simulink model "TST_AccPed_DoCoordOut"  (R2016b)
settings: Solver=FixedStepDiscrete  StartTime=0.0  StopTime=simTime  FixedStep=sampleTime  RelTol=1e-3
values from neighbouring files (symbols this model uses):
  testCase = 1    [initTST_AccPed_DoCoordOut_001.m]    (also in initTST_AccPed_DoCoordOut_002.m = 2; initTST_AccPed_DoCoordOut_003.m = 3)
libraries: simulink x31, UnitTest_Lib x27
settings Model: Creator=zhengjinyan  LastModifiedBy=zhengjinyan
settings DebuggingCC: SignalRangeChecking=error

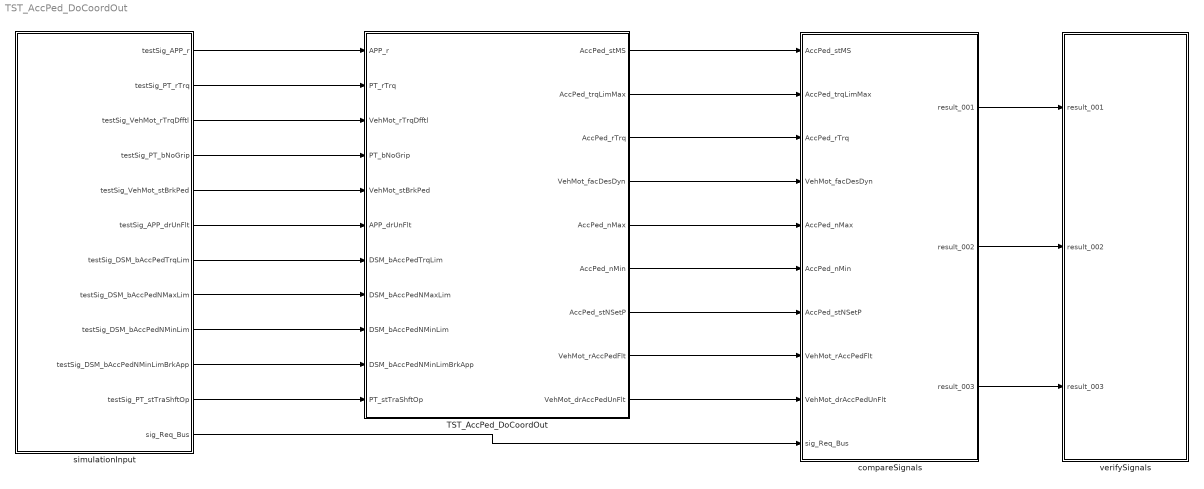
== system TST_AccPed_DoCoordOut ==
  TST_AccPed_DoCoordOut : Subsystem
  compareSignals : Subsystem
  simulationInput : Subsystem
  verifySignals : Subsystem
  wires:
  simulationInput/1(testSig_APP_r) -> TST_AccPed_DoCoordOut/1(APP_r)
  simulationInput/2(testSig_PT_rTrq) -> TST_AccPed_DoCoordOut/2(PT_rTrq)
  simulationInput/3(testSig_VehMot_rTrqDfftl) -> TST_AccPed_DoCoordOut/3(VehMot_rTrqDfftl)
  simulationInput/4(testSig_PT_bNoGrip) -> TST_AccPed_DoCoordOut/4(PT_bNoGrip)
  simulationInput/5(testSig_VehMot_stBrkPed) -> TST_AccPed_DoCoordOut/5(VehMot_stBrkPed)
  simulationInput/6(testSig_APP_drUnFlt) -> TST_AccPed_DoCoordOut/6(APP_drUnFlt)
  simulationInput/7(testSig_DSM_bAccPedTrqLim) -> TST_AccPed_DoCoordOut/7(DSM_bAccPedTrqLim)
  simulationInput/8(testSig_DSM_bAccPedNMaxLim) -> TST_AccPed_DoCoordOut/8(DSM_bAccPedNMaxLim)
  simulationInput/9(testSig_DSM_bAccPedNMinLim) -> TST_AccPed_DoCoordOut/9(DSM_bAccPedNMinLim)
  simulationInput/10(testSig_DSM_bAccPedNMinLimBrkApp) -> TST_AccPed_DoCoordOut/10(DSM_bAccPedNMinLimBrkApp)
  simulationInput/11(testSig_PT_stTraShftOp) -> TST_AccPed_DoCoordOut/11(PT_stTraShftOp)
  TST_AccPed_DoCoordOut/1(AccPed_stMS) -> compareSignals/1(AccPed_stMS)
  TST_AccPed_DoCoordOut/2(AccPed_trqLimMax) -> compareSignals/2(AccPed_trqLimMax)
  TST_AccPed_DoCoordOut/3(AccPed_rTrq) -> compareSignals/3(AccPed_rTrq)
  TST_AccPed_DoCoordOut/4(VehMot_facDesDyn) -> compareSignals/4(VehMot_facDesDyn)
  TST_AccPed_DoCoordOut/5(AccPed_nMax) -> compareSignals/5(AccPed_nMax)
  TST_AccPed_DoCoordOut/6(AccPed_nMin) -> compareSignals/6(AccPed_nMin)
  TST_AccPed_DoCoordOut/7(AccPed_stNSetP) -> compareSignals/7(AccPed_stNSetP)
  TST_AccPed_DoCoordOut/8(VehMot_rAccPedFlt) -> compareSignals/8(VehMot_rAccPedFlt)
  TST_AccPed_DoCoordOut/9(VehMot_drAccPedUnFlt) -> compareSignals/9(VehMot_drAccPedUnFlt)
  simulationInput/12(sig_Req_Bus) -> compareSignals/10(sig_Req_Bus)
  compareSignals/1(result_001) -> verifySignals/1(result_001)
  compareSignals/2(result_002) -> verifySignals/2(result_002)
  compareSignals/3(result_003) -> verifySignals/3(result_003)

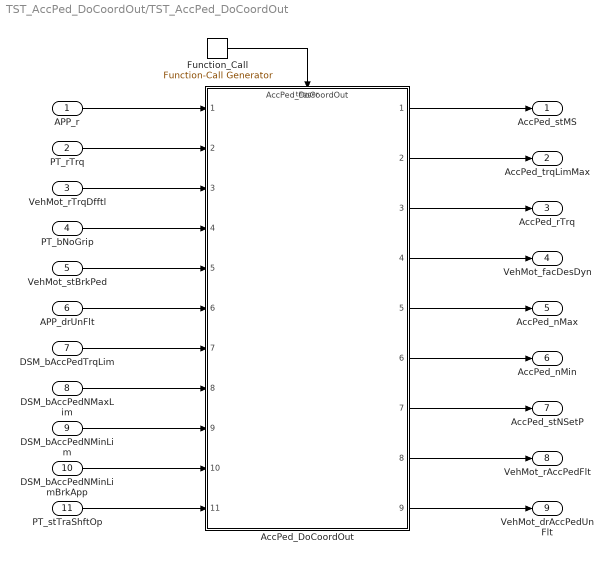
== system TST_AccPed_DoCoordOut/TST_AccPed_DoCoordOut ==
  APP_r : Inport
  PT_rTrq : Inport  Port=2
  VehMot_rTrqDfftl : Inport  Port=3
  PT_bNoGrip : Inport  Port=4
  VehMot_stBrkPed : Inport  Port=5
  APP_drUnFlt : Inport  Port=6
  DSM_bAccPedTrqLim : Inport  Port=7
  DSM_bAccPedNMaxLim : Inport  Port=8
  DSM_bAccPedNMinLim : Inport  Port=9
  DSM_bAccPedNMinLimBrkApp : Inport  Port=10
  PT_stTraShftOp : Inport  Port=11
  AccPed_DoCoordOut : ModelReference  ModelNameDialog=AccPed_DoCoordOut  SimulationMode=Normal  ModelReferenceVersion=1.27  TriggerPortName=function  TriggerPortTriggerType=function-call  TriggerPortStatesWhenEnabling=held
  Function_Call : simulink/Ports & Subsystems/Function-Call Generator  sample_time=sampleTime  numberOfIterations=1
  AccPed_stMS : Outport
  AccPed_trqLimMax : Outport  Port=2
  AccPed_rTrq : Outport  Port=3
  VehMot_facDesDyn : Outport  Port=4
  AccPed_nMax : Outport  Port=5
  AccPed_nMin : Outport  Port=6
  AccPed_stNSetP : Outport  Port=7
  VehMot_rAccPedFlt : Outport  Port=8
  VehMot_drAccPedUnFlt : Outport  Port=9
  wires:
  Function_Call/1 -> AccPed_DoCoordOut/Trigger
  APP_r/1 -> AccPed_DoCoordOut/1
  PT_rTrq/1 -> AccPed_DoCoordOut/2
  VehMot_rTrqDfftl/1 -> AccPed_DoCoordOut/3
  PT_bNoGrip/1 -> AccPed_DoCoordOut/4
  VehMot_stBrkPed/1 -> AccPed_DoCoordOut/5
  APP_drUnFlt/1 -> AccPed_DoCoordOut/6
  DSM_bAccPedTrqLim/1 -> AccPed_DoCoordOut/7
  DSM_bAccPedNMaxLim/1 -> AccPed_DoCoordOut/8
  DSM_bAccPedNMinLim/1 -> AccPed_DoCoordOut/9
  DSM_bAccPedNMinLimBrkApp/1 -> AccPed_DoCoordOut/10
  PT_stTraShftOp/1 -> AccPed_DoCoordOut/11
  AccPed_DoCoordOut/1 -> AccPed_stMS/1
  AccPed_DoCoordOut/2 -> AccPed_trqLimMax/1
  AccPed_DoCoordOut/3 -> AccPed_rTrq/1
  AccPed_DoCoordOut/4 -> VehMot_facDesDyn/1
  AccPed_DoCoordOut/5 -> AccPed_nMax/1
  AccPed_DoCoordOut/6 -> AccPed_nMin/1
  AccPed_DoCoordOut/7 -> AccPed_stNSetP/1
  AccPed_DoCoordOut/8 -> VehMot_rAccPedFlt/1
  AccPed_DoCoordOut/9 -> VehMot_drAccPedUnFlt/1

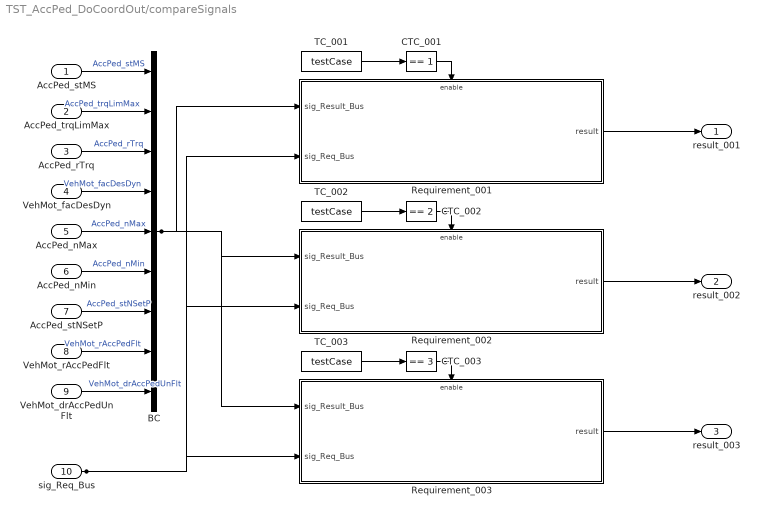
== system TST_AccPed_DoCoordOut/compareSignals ==
  AccPed_stMS : Inport
  AccPed_trqLimMax : Inport  Port=2
  AccPed_rTrq : Inport  Port=3
  VehMot_facDesDyn : Inport  Port=4
  AccPed_nMax : Inport  Port=5
  AccPed_nMin : Inport  Port=6
  AccPed_stNSetP : Inport  Port=7
  VehMot_rAccPedFlt : Inport  Port=8
  VehMot_drAccPedUnFlt : Inport  Port=9
  sig_Req_Bus : Inport  Port=10
  BC : BusCreator  Inputs=9
  CTC_001 : simulink/Logic and Bit Operations/Compare To Constant  relop===  const=1  OutDataTypeStr=boolean
  CTC_002 : simulink/Logic and Bit Operations/Compare To Constant  relop===  const=2  OutDataTypeStr=boolean
  CTC_003 : simulink/Logic and Bit Operations/Compare To Constant  relop===  const=3  OutDataTypeStr=boolean
  Requirement_001 : Subsystem
  Requirement_002 : Subsystem
  Requirement_003 : Subsystem
  TC_001 : Constant  Value=testCase
  TC_002 : Constant  Value=testCase
  TC_003 : Constant  Value=testCase
  result_001 : Outport
  result_002 : Outport  Port=2
  result_003 : Outport  Port=3
  wires:
  AccPed_stMS/1 -> BC/1  "AccPed_stMS"
  AccPed_trqLimMax/1 -> BC/2  "AccPed_trqLimMax"
  AccPed_rTrq/1 -> BC/3  "AccPed_rTrq"
  VehMot_facDesDyn/1 -> BC/4  "VehMot_facDesDyn"
  AccPed_nMax/1 -> BC/5  "AccPed_nMax"
  AccPed_nMin/1 -> BC/6  "AccPed_nMin"
  AccPed_stNSetP/1 -> BC/7  "AccPed_stNSetP"
  VehMot_rAccPedFlt/1 -> BC/8  "VehMot_rAccPedFlt"
  VehMot_drAccPedUnFlt/1 -> BC/9  "VehMot_drAccPedUnFlt"
  TC_001/1 -> CTC_001/1
  CTC_001/1 -> Requirement_001/Enable
  sig_Req_Bus/1 -> Requirement_001/2(sig_Req_Bus), Requirement_002/2(sig_Req_Bus), Requirement_003/2(sig_Req_Bus)
  BC/1 -> Requirement_001/1(sig_Result_Bus), Requirement_002/1(sig_Result_Bus), Requirement_003/1(sig_Result_Bus)
  Requirement_001/1(result) -> result_001/1
  TC_002/1 -> CTC_002/1
  CTC_002/1 -> Requirement_002/Enable
  Requirement_002/1(result) -> result_002/1
  TC_003/1 -> CTC_003/1
  CTC_003/1 -> Requirement_003/Enable
  Requirement_003/1(result) -> result_003/1

== system TST_AccPed_DoCoordOut/simulationInput ==
  BS : BusSelector  OutputSignals=testSig_APP_r,testSig_PT_rTrq,testSig_VehMot_rTrqDfftl,testSig_PT_bNoGrip,testSig_VehMot_stBrkPed,testSig_APP_drUnFlt,testSig_DSM_bAccPedTrqLim,testSig_DSM_bAccPedNMaxLim,testSig_DSM_bAccPedNMinLim,testSig_DSM_bAccPedNMinLimBrkApp,testSig_PT_stTraShftOp
  MPSw : MultiPortSwitch  SaturateOnIntegerOverflow=on  InputSameDT=on
  TestCase : Constant  Value=testCase
  testSignals_R001 : Subsystem
  testSignals_R002 : Subsystem
  testSignals_R003 : Subsystem
  testSig_APP_r : Outport
  testSig_PT_rTrq : Outport  Port=2
  testSig_VehMot_rTrqDfftl : Outport  Port=3
  testSig_PT_bNoGrip : Outport  Port=4
  testSig_VehMot_stBrkPed : Outport  Port=5
  testSig_APP_drUnFlt : Outport  Port=6
  testSig_DSM_bAccPedTrqLim : Outport  Port=7
  testSig_DSM_bAccPedNMaxLim : Outport  Port=8
  testSig_DSM_bAccPedNMinLim : Outport  Port=9
  testSig_DSM_bAccPedNMinLimBrkApp : Outport  Port=10
  testSig_PT_stTraShftOp : Outport  Port=11
  sig_Req_Bus : Outport  Port=12
  wires:
  BS/1 -> testSig_APP_r/1  "<testSig_APP_r>"
  BS/2 -> testSig_PT_rTrq/1  "<testSig_PT_rTrq>"
  BS/3 -> testSig_VehMot_rTrqDfftl/1  "<testSig_VehMot_rTrqDfftl>"
  BS/4 -> testSig_PT_bNoGrip/1  "<testSig_PT_bNoGrip>"
  BS/5 -> testSig_VehMot_stBrkPed/1  "<testSig_VehMot_stBrkPed>"
  BS/6 -> testSig_APP_drUnFlt/1  "<testSig_APP_drUnFlt>"
  BS/7 -> testSig_DSM_bAccPedTrqLim/1  "<testSig_DSM_bAccPedTrqLim>"
  BS/8 -> testSig_DSM_bAccPedNMaxLim/1  "<testSig_DSM_bAccPedNMaxLim>"
  BS/9 -> testSig_DSM_bAccPedNMinLim/1  "<testSig_DSM_bAccPedNMinLim>"
  BS/10 -> testSig_DSM_bAccPedNMinLimBrkApp/1  "<testSig_DSM_bAccPedNMinLimBrkApp>"
  BS/11 -> testSig_PT_stTraShftOp/1  "<testSig_PT_stTraShftOp>"
  MPSw/1 -> BS/1, sig_Req_Bus/1
  TestCase/1 -> MPSw/1
  testSignals_R001/1(testSignals) -> MPSw/2
  testSignals_R002/1(testSignals) -> MPSw/3
  testSignals_R003/1(testSignals) -> MPSw/4

== system TST_AccPed_DoCoordOut/verifySignals ==
  result_001 : Inport
  result_002 : Inport  Port=2
  result_003 : Inport  Port=3
  Assertion_001 : Assertion  Enabled=off
  Assertion_002 : Assertion  Enabled=off
  Assertion_003 : Assertion  Enabled=off
  wires:
  result_001/1 -> Assertion_001/1
  result_002/1 -> Assertion_002/1
  result_003/1 -> Assertion_003/1

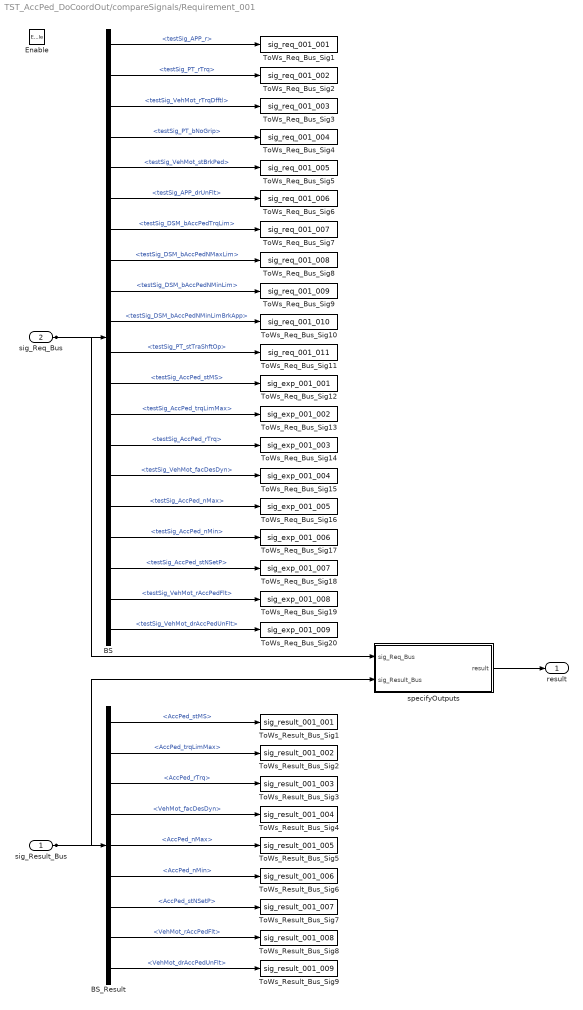
== system TST_AccPed_DoCoordOut/compareSignals/Requirement_001 ==
  sig_Result_Bus : Inport
  sig_Req_Bus : Inport  Port=2
  Enable : EnablePort
  BS : BusSelector  OutputSignals=testSig_APP_r,testSig_PT_rTrq,testSig_VehMot_rTrqDfftl,testSig_PT_bNoGrip,testSig_VehMot_stBrkPed,testSig_APP_drUnFlt,testSig_DSM_bAccPedTrqLim,testSig_DSM_bAccPedNMaxLim,testSig_DSM_bAccPedNMinLim,testSig_DSM_bAccPedNMinLimBrkApp,testSig_PT_stTraShftOp,testSig_AccPed_stMS,testSig_AccPed_trqLimMax,testSig_AccPed_rTrq,testSig_VehMot_facDesDyn,testSig_AccPed_nMax,testSig_AccPed_nMin,testSig_AccPed_stNSetP,testSig_VehMot_rAccPedFlt,testSig_VehMot_drAccPedUnFlt
  BS_Result : BusSelector  OutputSignals=AccPed_stMS,AccPed_trqLimMax,AccPed_rTrq,VehMot_facDesDyn,AccPed_nMax,AccPed_nMin,AccPed_stNSetP,VehMot_rAccPedFlt,VehMot_drAccPedUnFlt
  ToWs_Req_Bus_Sig1 : ToWorkspace  VariableName=sig_req_001_001  SaveFormat=Structure With Time
  ToWs_Req_Bus_Sig10 : ToWorkspace  VariableName=sig_req_001_010  SaveFormat=Structure With Time
  ToWs_Req_Bus_Sig11 : ToWorkspace  VariableName=sig_req_001_011  SaveFormat=Structure With Time
  ToWs_Req_Bus_Sig12 : ToWorkspace  VariableName=sig_exp_001_001  SaveFormat=Structure With Time
  ToWs_Req_Bus_Sig13 : ToWorkspace  VariableName=sig_exp_001_002  SaveFormat=Structure With Time
  ToWs_Req_Bus_Sig14 : ToWorkspace  VariableName=sig_exp_001_003  SaveFormat=Structure With Time
  ToWs_Req_Bus_Sig15 : ToWorkspace  VariableName=sig_exp_001_004  SaveFormat=Structure With Time
  ToWs_Req_Bus_Sig16 : ToWorkspace  VariableName=sig_exp_001_005  SaveFormat=Structure With Time
  ToWs_Req_Bus_Sig17 : ToWorkspace  VariableName=sig_exp_001_006  SaveFormat=Structure With Time
  ToWs_Req_Bus_Sig18 : ToWorkspace  VariableName=sig_exp_001_007  SaveFormat=Structure With Time
  ToWs_Req_Bus_Sig19 : ToWorkspace  VariableName=sig_exp_001_008  SaveFormat=Structure With Time
  ToWs_Req_Bus_Sig2 : ToWorkspace  VariableName=sig_req_001_002  SaveFormat=Structure With Time
  ToWs_Req_Bus_Sig20 : ToWorkspace  VariableName=sig_exp_001_009  SaveFormat=Structure With Time
  ToWs_Req_Bus_Sig3 : ToWorkspace  VariableName=sig_req_001_003  SaveFormat=Structure With Time
  ToWs_Req_Bus_Sig4 : ToWorkspace  VariableName=sig_req_001_004  SaveFormat=Structure With Time
  ToWs_Req_Bus_Sig5 : ToWorkspace  VariableName=sig_req_001_005  SaveFormat=Structure With Time
  ToWs_Req_Bus_Sig6 : ToWorkspace  VariableName=sig_req_001_006  SaveFormat=Structure With Time
  ToWs_Req_Bus_Sig7 : ToWorkspace  VariableName=sig_req_001_007  SaveFormat=Structure With Time
  ToWs_Req_Bus_Sig8 : ToWorkspace  VariableName=sig_req_001_008  SaveFormat=Structure With Time
  ToWs_Req_Bus_Sig9 : ToWorkspace  VariableName=sig_req_001_009  SaveFormat=Structure With Time
  ToWs_Result_Bus_Sig1 : ToWorkspace  VariableName=sig_result_001_001  SaveFormat=Structure With Time
  ToWs_Result_Bus_Sig2 : ToWorkspace  VariableName=sig_result_001_002  SaveFormat=Structure With Time
  ToWs_Result_Bus_Sig3 : ToWorkspace  VariableName=sig_result_001_003  SaveFormat=Structure With Time
  ToWs_Result_Bus_Sig4 : ToWorkspace  VariableName=sig_result_001_004  SaveFormat=Structure With Time
  ToWs_Result_Bus_Sig5 : ToWorkspace  VariableName=sig_result_001_005  SaveFormat=Structure With Time
  ToWs_Result_Bus_Sig6 : ToWorkspace  VariableName=sig_result_001_006  SaveFormat=Structure With Time
  ToWs_Result_Bus_Sig7 : ToWorkspace  VariableName=sig_result_001_007  SaveFormat=Structure With Time
  ToWs_Result_Bus_Sig8 : ToWorkspace  VariableName=sig_result_001_008  SaveFormat=Structure With Time
  ToWs_Result_Bus_Sig9 : ToWorkspace  VariableName=sig_result_001_009  SaveFormat=Structure With Time
  specifyOutputs : Subsystem
  result : Outport
  wires:
  sig_Req_Bus/1 -> BS/1, specifyOutputs/1(sig_Req_Bus)
  BS/1 -> ToWs_Req_Bus_Sig1/1  "<testSig_APP_r>"
  BS/2 -> ToWs_Req_Bus_Sig2/1  "<testSig_PT_rTrq>"
  BS/3 -> ToWs_Req_Bus_Sig3/1  "<testSig_VehMot_rTrqDfftl>"
  BS/4 -> ToWs_Req_Bus_Sig4/1  "<testSig_PT_bNoGrip>"
  BS/5 -> ToWs_Req_Bus_Sig5/1  "<testSig_VehMot_stBrkPed>"
  BS/6 -> ToWs_Req_Bus_Sig6/1  "<testSig_APP_drUnFlt>"
  BS/7 -> ToWs_Req_Bus_Sig7/1  "<testSig_DSM_bAccPedTrqLim>"
  BS/8 -> ToWs_Req_Bus_Sig8/1  "<testSig_DSM_bAccPedNMaxLim>"
  BS/9 -> ToWs_Req_Bus_Sig9/1  "<testSig_DSM_bAccPedNMinLim>"
  BS/10 -> ToWs_Req_Bus_Sig10/1  "<testSig_DSM_bAccPedNMinLimBrkApp>"
  BS/11 -> ToWs_Req_Bus_Sig11/1  "<testSig_PT_stTraShftOp>"
  BS/12 -> ToWs_Req_Bus_Sig12/1  "<testSig_AccPed_stMS>"
  BS/13 -> ToWs_Req_Bus_Sig13/1  "<testSig_AccPed_trqLimMax>"
  BS/14 -> ToWs_Req_Bus_Sig14/1  "<testSig_AccPed_rTrq>"
  BS/15 -> ToWs_Req_Bus_Sig15/1  "<testSig_VehMot_facDesDyn>"
  BS/16 -> ToWs_Req_Bus_Sig16/1  "<testSig_AccPed_nMax>"
  BS/17 -> ToWs_Req_Bus_Sig17/1  "<testSig_AccPed_nMin>"
  BS/18 -> ToWs_Req_Bus_Sig18/1  "<testSig_AccPed_stNSetP>"
  BS/19 -> ToWs_Req_Bus_Sig19/1  "<testSig_VehMot_rAccPedFlt>"
  BS/20 -> ToWs_Req_Bus_Sig20/1  "<testSig_VehMot_drAccPedUnFlt>"
  sig_Result_Bus/1 -> BS_Result/1, specifyOutputs/2(sig_Result_Bus)
  BS_Result/1 -> ToWs_Result_Bus_Sig1/1  "<AccPed_stMS>"
  BS_Result/2 -> ToWs_Result_Bus_Sig2/1  "<AccPed_trqLimMax>"
  BS_Result/3 -> ToWs_Result_Bus_Sig3/1  "<AccPed_rTrq>"
  BS_Result/4 -> ToWs_Result_Bus_Sig4/1  "<VehMot_facDesDyn>"
  BS_Result/5 -> ToWs_Result_Bus_Sig5/1  "<AccPed_nMax>"
  BS_Result/6 -> ToWs_Result_Bus_Sig6/1  "<AccPed_nMin>"
  BS_Result/7 -> ToWs_Result_Bus_Sig7/1  "<AccPed_stNSetP>"
  BS_Result/8 -> ToWs_Result_Bus_Sig8/1  "<VehMot_rAccPedFlt>"
  BS_Result/9 -> ToWs_Result_Bus_Sig9/1  "<VehMot_drAccPedUnFlt>"
  specifyOutputs/1(result) -> result/1

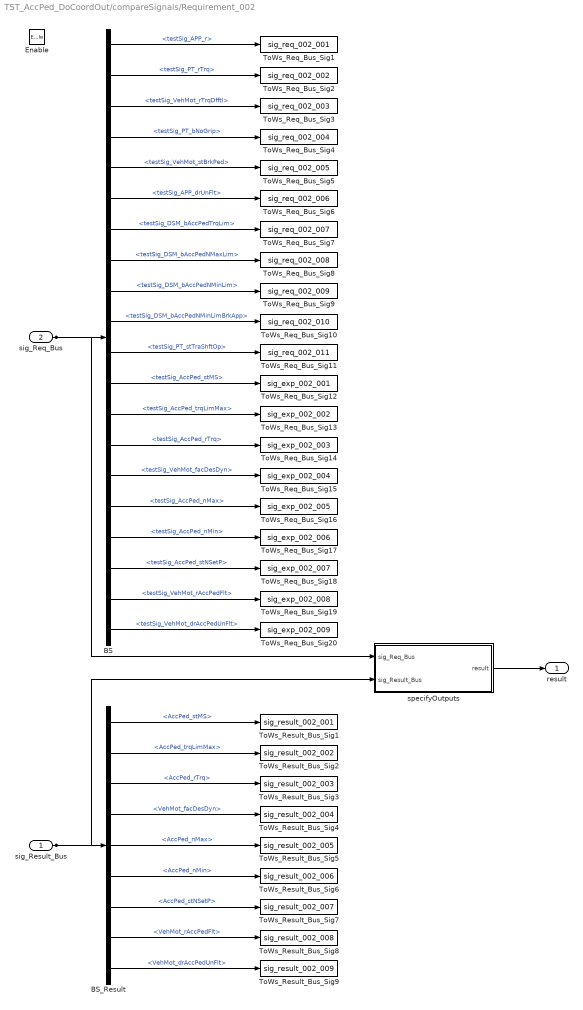
== system TST_AccPed_DoCoordOut/compareSignals/Requirement_002 ==
  sig_Result_Bus : Inport
  sig_Req_Bus : Inport  Port=2
  Enable : EnablePort
  BS : BusSelector  OutputSignals=testSig_APP_r,testSig_PT_rTrq,testSig_VehMot_rTrqDfftl,testSig_PT_bNoGrip,testSig_VehMot_stBrkPed,testSig_APP_drUnFlt,testSig_DSM_bAccPedTrqLim,testSig_DSM_bAccPedNMaxLim,testSig_DSM_bAccPedNMinLim,testSig_DSM_bAccPedNMinLimBrkApp,testSig_PT_stTraShftOp,testSig_AccPed_stMS,testSig_AccPed_trqLimMax,testSig_AccPed_rTrq,testSig_VehMot_facDesDyn,testSig_AccPed_nMax,testSig_AccPed_nMin,testSig_AccPed_stNSetP,testSig_VehMot_rAccPedFlt,testSig_VehMot_drAccPedUnFlt
  BS_Result : BusSelector  OutputSignals=AccPed_stMS,AccPed_trqLimMax,AccPed_rTrq,VehMot_facDesDyn,AccPed_nMax,AccPed_nMin,AccPed_stNSetP,VehMot_rAccPedFlt,VehMot_drAccPedUnFlt
  ToWs_Req_Bus_Sig1 : ToWorkspace  VariableName=sig_req_002_001  SaveFormat=Structure With Time
  ToWs_Req_Bus_Sig10 : ToWorkspace  VariableName=sig_req_002_010  SaveFormat=Structure With Time
  ToWs_Req_Bus_Sig11 : ToWorkspace  VariableName=sig_req_002_011  SaveFormat=Structure With Time
  ToWs_Req_Bus_Sig12 : ToWorkspace  VariableName=sig_exp_002_001  SaveFormat=Structure With Time
  ToWs_Req_Bus_Sig13 : ToWorkspace  VariableName=sig_exp_002_002  SaveFormat=Structure With Time
  ToWs_Req_Bus_Sig14 : ToWorkspace  VariableName=sig_exp_002_003  SaveFormat=Structure With Time
  ToWs_Req_Bus_Sig15 : ToWorkspace  VariableName=sig_exp_002_004  SaveFormat=Structure With Time
  ToWs_Req_Bus_Sig16 : ToWorkspace  VariableName=sig_exp_002_005  SaveFormat=Structure With Time
  ToWs_Req_Bus_Sig17 : ToWorkspace  VariableName=sig_exp_002_006  SaveFormat=Structure With Time
  ToWs_Req_Bus_Sig18 : ToWorkspace  VariableName=sig_exp_002_007  SaveFormat=Structure With Time
  ToWs_Req_Bus_Sig19 : ToWorkspace  VariableName=sig_exp_002_008  SaveFormat=Structure With Time
  ToWs_Req_Bus_Sig2 : ToWorkspace  VariableName=sig_req_002_002  SaveFormat=Structure With Time
  ToWs_Req_Bus_Sig20 : ToWorkspace  VariableName=sig_exp_002_009  SaveFormat=Structure With Time
  ToWs_Req_Bus_Sig3 : ToWorkspace  VariableName=sig_req_002_003  SaveFormat=Structure With Time
  ToWs_Req_Bus_Sig4 : ToWorkspace  VariableName=sig_req_002_004  SaveFormat=Structure With Time
  ToWs_Req_Bus_Sig5 : ToWorkspace  VariableName=sig_req_002_005  SaveFormat=Structure With Time
  ToWs_Req_Bus_Sig6 : ToWorkspace  VariableName=sig_req_002_006  SaveFormat=Structure With Time
  ToWs_Req_Bus_Sig7 : ToWorkspace  VariableName=sig_req_002_007  SaveFormat=Structure With Time
  ToWs_Req_Bus_Sig8 : ToWorkspace  VariableName=sig_req_002_008  SaveFormat=Structure With Time
  ToWs_Req_Bus_Sig9 : ToWorkspace  VariableName=sig_req_002_009  SaveFormat=Structure With Time
  ToWs_Result_Bus_Sig1 : ToWorkspace  VariableName=sig_result_002_001  SaveFormat=Structure With Time
  ToWs_Result_Bus_Sig2 : ToWorkspace  VariableName=sig_result_002_002  SaveFormat=Structure With Time
  ToWs_Result_Bus_Sig3 : ToWorkspace  VariableName=sig_result_002_003  SaveFormat=Structure With Time
  ToWs_Result_Bus_Sig4 : ToWorkspace  VariableName=sig_result_002_004  SaveFormat=Structure With Time
  ToWs_Result_Bus_Sig5 : ToWorkspace  VariableName=sig_result_002_005  SaveFormat=Structure With Time
  ToWs_Result_Bus_Sig6 : ToWorkspace  VariableName=sig_result_002_006  SaveFormat=Structure With Time
  ToWs_Result_Bus_Sig7 : ToWorkspace  VariableName=sig_result_002_007  SaveFormat=Structure With Time
  ToWs_Result_Bus_Sig8 : ToWorkspace  VariableName=sig_result_002_008  SaveFormat=Structure With Time
  ToWs_Result_Bus_Sig9 : ToWorkspace  VariableName=sig_result_002_009  SaveFormat=Structure With Time
  specifyOutputs : Subsystem
  result : Outport
  wires:
  sig_Req_Bus/1 -> BS/1, specifyOutputs/1(sig_Req_Bus)
  BS/1 -> ToWs_Req_Bus_Sig1/1  "<testSig_APP_r>"
  BS/2 -> ToWs_Req_Bus_Sig2/1  "<testSig_PT_rTrq>"
  BS/3 -> ToWs_Req_Bus_Sig3/1  "<testSig_VehMot_rTrqDfftl>"
  BS/4 -> ToWs_Req_Bus_Sig4/1  "<testSig_PT_bNoGrip>"
  BS/5 -> ToWs_Req_Bus_Sig5/1  "<testSig_VehMot_stBrkPed>"
  BS/6 -> ToWs_Req_Bus_Sig6/1  "<testSig_APP_drUnFlt>"
  BS/7 -> ToWs_Req_Bus_Sig7/1  "<testSig_DSM_bAccPedTrqLim>"
  BS/8 -> ToWs_Req_Bus_Sig8/1  "<testSig_DSM_bAccPedNMaxLim>"
  BS/9 -> ToWs_Req_Bus_Sig9/1  "<testSig_DSM_bAccPedNMinLim>"
  BS/10 -> ToWs_Req_Bus_Sig10/1  "<testSig_DSM_bAccPedNMinLimBrkApp>"
  BS/11 -> ToWs_Req_Bus_Sig11/1  "<testSig_PT_stTraShftOp>"
  BS/12 -> ToWs_Req_Bus_Sig12/1  "<testSig_AccPed_stMS>"
  BS/13 -> ToWs_Req_Bus_Sig13/1  "<testSig_AccPed_trqLimMax>"
  BS/14 -> ToWs_Req_Bus_Sig14/1  "<testSig_AccPed_rTrq>"
  BS/15 -> ToWs_Req_Bus_Sig15/1  "<testSig_VehMot_facDesDyn>"
  BS/16 -> ToWs_Req_Bus_Sig16/1  "<testSig_AccPed_nMax>"
  BS/17 -> ToWs_Req_Bus_Sig17/1  "<testSig_AccPed_nMin>"
  BS/18 -> ToWs_Req_Bus_Sig18/1  "<testSig_AccPed_stNSetP>"
  BS/19 -> ToWs_Req_Bus_Sig19/1  "<testSig_VehMot_rAccPedFlt>"
  BS/20 -> ToWs_Req_Bus_Sig20/1  "<testSig_VehMot_drAccPedUnFlt>"
  sig_Result_Bus/1 -> BS_Result/1, specifyOutputs/2(sig_Result_Bus)
  BS_Result/1 -> ToWs_Result_Bus_Sig1/1  "<AccPed_stMS>"
  BS_Result/2 -> ToWs_Result_Bus_Sig2/1  "<AccPed_trqLimMax>"
  BS_Result/3 -> ToWs_Result_Bus_Sig3/1  "<AccPed_rTrq>"
  BS_Result/4 -> ToWs_Result_Bus_Sig4/1  "<VehMot_facDesDyn>"
  BS_Result/5 -> ToWs_Result_Bus_Sig5/1  "<AccPed_nMax>"
  BS_Result/6 -> ToWs_Result_Bus_Sig6/1  "<AccPed_nMin>"
  BS_Result/7 -> ToWs_Result_Bus_Sig7/1  "<AccPed_stNSetP>"
  BS_Result/8 -> ToWs_Result_Bus_Sig8/1  "<VehMot_rAccPedFlt>"
  BS_Result/9 -> ToWs_Result_Bus_Sig9/1  "<VehMot_drAccPedUnFlt>"
  specifyOutputs/1(result) -> result/1

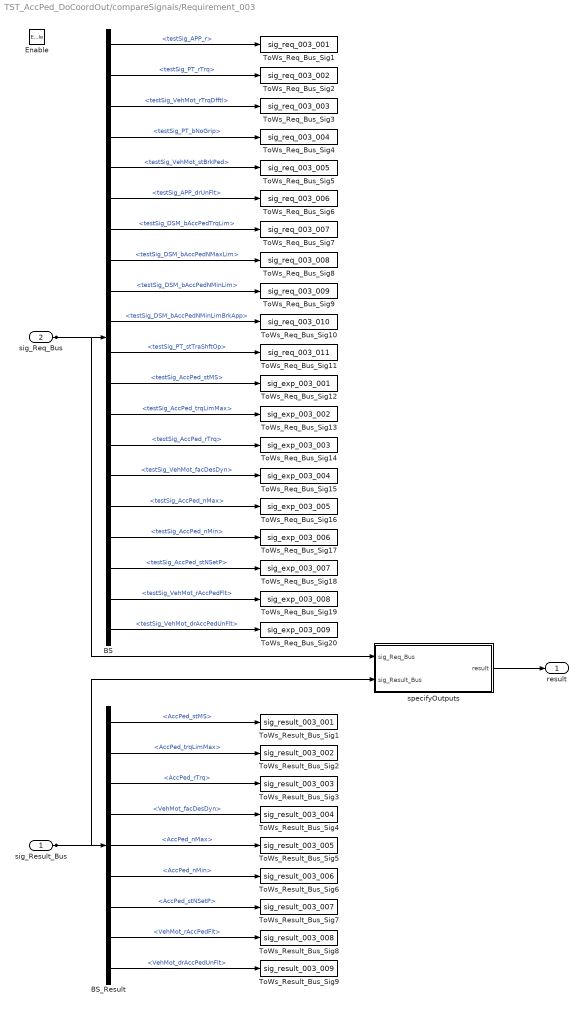
== system TST_AccPed_DoCoordOut/compareSignals/Requirement_003 ==
  sig_Result_Bus : Inport
  sig_Req_Bus : Inport  Port=2
  Enable : EnablePort
  BS : BusSelector  OutputSignals=testSig_APP_r,testSig_PT_rTrq,testSig_VehMot_rTrqDfftl,testSig_PT_bNoGrip,testSig_VehMot_stBrkPed,testSig_APP_drUnFlt,testSig_DSM_bAccPedTrqLim,testSig_DSM_bAccPedNMaxLim,testSig_DSM_bAccPedNMinLim,testSig_DSM_bAccPedNMinLimBrkApp,testSig_PT_stTraShftOp,testSig_AccPed_stMS,testSig_AccPed_trqLimMax,testSig_AccPed_rTrq,testSig_VehMot_facDesDyn,testSig_AccPed_nMax,testSig_AccPed_nMin,testSig_AccPed_stNSetP,testSig_VehMot_rAccPedFlt,testSig_VehMot_drAccPedUnFlt
  BS_Result : BusSelector  OutputSignals=AccPed_stMS,AccPed_trqLimMax,AccPed_rTrq,VehMot_facDesDyn,AccPed_nMax,AccPed_nMin,AccPed_stNSetP,VehMot_rAccPedFlt,VehMot_drAccPedUnFlt
  ToWs_Req_Bus_Sig1 : ToWorkspace  VariableName=sig_req_003_001  SaveFormat=Structure With Time
  ToWs_Req_Bus_Sig10 : ToWorkspace  VariableName=sig_req_003_010  SaveFormat=Structure With Time
  ToWs_Req_Bus_Sig11 : ToWorkspace  VariableName=sig_req_003_011  SaveFormat=Structure With Time
  ToWs_Req_Bus_Sig12 : ToWorkspace  VariableName=sig_exp_003_001  SaveFormat=Structure With Time
  ToWs_Req_Bus_Sig13 : ToWorkspace  VariableName=sig_exp_003_002  SaveFormat=Structure With Time
  ToWs_Req_Bus_Sig14 : ToWorkspace  VariableName=sig_exp_003_003  SaveFormat=Structure With Time
  ToWs_Req_Bus_Sig15 : ToWorkspace  VariableName=sig_exp_003_004  SaveFormat=Structure With Time
  ToWs_Req_Bus_Sig16 : ToWorkspace  VariableName=sig_exp_003_005  SaveFormat=Structure With Time
  ToWs_Req_Bus_Sig17 : ToWorkspace  VariableName=sig_exp_003_006  SaveFormat=Structure With Time
  ToWs_Req_Bus_Sig18 : ToWorkspace  VariableName=sig_exp_003_007  SaveFormat=Structure With Time
  ToWs_Req_Bus_Sig19 : ToWorkspace  VariableName=sig_exp_003_008  SaveFormat=Structure With Time
  ToWs_Req_Bus_Sig2 : ToWorkspace  VariableName=sig_req_003_002  SaveFormat=Structure With Time
  ToWs_Req_Bus_Sig20 : ToWorkspace  VariableName=sig_exp_003_009  SaveFormat=Structure With Time
  ToWs_Req_Bus_Sig3 : ToWorkspace  VariableName=sig_req_003_003  SaveFormat=Structure With Time
  ToWs_Req_Bus_Sig4 : ToWorkspace  VariableName=sig_req_003_004  SaveFormat=Structure With Time
  ToWs_Req_Bus_Sig5 : ToWorkspace  VariableName=sig_req_003_005  SaveFormat=Structure With Time
  ToWs_Req_Bus_Sig6 : ToWorkspace  VariableName=sig_req_003_006  SaveFormat=Structure With Time
  ToWs_Req_Bus_Sig7 : ToWorkspace  VariableName=sig_req_003_007  SaveFormat=Structure With Time
  ToWs_Req_Bus_Sig8 : ToWorkspace  VariableName=sig_req_003_008  SaveFormat=Structure With Time
  ToWs_Req_Bus_Sig9 : ToWorkspace  VariableName=sig_req_003_009  SaveFormat=Structure With Time
  ToWs_Result_Bus_Sig1 : ToWorkspace  VariableName=sig_result_003_001  SaveFormat=Structure With Time
  ToWs_Result_Bus_Sig2 : ToWorkspace  VariableName=sig_result_003_002  SaveFormat=Structure With Time
  ToWs_Result_Bus_Sig3 : ToWorkspace  VariableName=sig_result_003_003  SaveFormat=Structure With Time
  ToWs_Result_Bus_Sig4 : ToWorkspace  VariableName=sig_result_003_004  SaveFormat=Structure With Time
  ToWs_Result_Bus_Sig5 : ToWorkspace  VariableName=sig_result_003_005  SaveFormat=Structure With Time
  ToWs_Result_Bus_Sig6 : ToWorkspace  VariableName=sig_result_003_006  SaveFormat=Structure With Time
  ToWs_Result_Bus_Sig7 : ToWorkspace  VariableName=sig_result_003_007  SaveFormat=Structure With Time
  ToWs_Result_Bus_Sig8 : ToWorkspace  VariableName=sig_result_003_008  SaveFormat=Structure With Time
  ToWs_Result_Bus_Sig9 : ToWorkspace  VariableName=sig_result_003_009  SaveFormat=Structure With Time
  specifyOutputs : Subsystem
  result : Outport
  wires:
  sig_Req_Bus/1 -> BS/1, specifyOutputs/1(sig_Req_Bus)
  BS/1 -> ToWs_Req_Bus_Sig1/1  "<testSig_APP_r>"
  BS/2 -> ToWs_Req_Bus_Sig2/1  "<testSig_PT_rTrq>"
  BS/3 -> ToWs_Req_Bus_Sig3/1  "<testSig_VehMot_rTrqDfftl>"
  BS/4 -> ToWs_Req_Bus_Sig4/1  "<testSig_PT_bNoGrip>"
  BS/5 -> ToWs_Req_Bus_Sig5/1  "<testSig_VehMot_stBrkPed>"
  BS/6 -> ToWs_Req_Bus_Sig6/1  "<testSig_APP_drUnFlt>"
  BS/7 -> ToWs_Req_Bus_Sig7/1  "<testSig_DSM_bAccPedTrqLim>"
  BS/8 -> ToWs_Req_Bus_Sig8/1  "<testSig_DSM_bAccPedNMaxLim>"
  BS/9 -> ToWs_Req_Bus_Sig9/1  "<testSig_DSM_bAccPedNMinLim>"
  BS/10 -> ToWs_Req_Bus_Sig10/1  "<testSig_DSM_bAccPedNMinLimBrkApp>"
  BS/11 -> ToWs_Req_Bus_Sig11/1  "<testSig_PT_stTraShftOp>"
  BS/12 -> ToWs_Req_Bus_Sig12/1  "<testSig_AccPed_stMS>"
  BS/13 -> ToWs_Req_Bus_Sig13/1  "<testSig_AccPed_trqLimMax>"
  BS/14 -> ToWs_Req_Bus_Sig14/1  "<testSig_AccPed_rTrq>"
  BS/15 -> ToWs_Req_Bus_Sig15/1  "<testSig_VehMot_facDesDyn>"
  BS/16 -> ToWs_Req_Bus_Sig16/1  "<testSig_AccPed_nMax>"
  BS/17 -> ToWs_Req_Bus_Sig17/1  "<testSig_AccPed_nMin>"
  BS/18 -> ToWs_Req_Bus_Sig18/1  "<testSig_AccPed_stNSetP>"
  BS/19 -> ToWs_Req_Bus_Sig19/1  "<testSig_VehMot_rAccPedFlt>"
  BS/20 -> ToWs_Req_Bus_Sig20/1  "<testSig_VehMot_drAccPedUnFlt>"
  sig_Result_Bus/1 -> BS_Result/1, specifyOutputs/2(sig_Result_Bus)
  BS_Result/1 -> ToWs_Result_Bus_Sig1/1  "<AccPed_stMS>"
  BS_Result/2 -> ToWs_Result_Bus_Sig2/1  "<AccPed_trqLimMax>"
  BS_Result/3 -> ToWs_Result_Bus_Sig3/1  "<AccPed_rTrq>"
  BS_Result/4 -> ToWs_Result_Bus_Sig4/1  "<VehMot_facDesDyn>"
  BS_Result/5 -> ToWs_Result_Bus_Sig5/1  "<AccPed_nMax>"
  BS_Result/6 -> ToWs_Result_Bus_Sig6/1  "<AccPed_nMin>"
  BS_Result/7 -> ToWs_Result_Bus_Sig7/1  "<AccPed_stNSetP>"
  BS_Result/8 -> ToWs_Result_Bus_Sig8/1  "<VehMot_rAccPedFlt>"
  BS_Result/9 -> ToWs_Result_Bus_Sig9/1  "<VehMot_drAccPedUnFlt>"
  specifyOutputs/1(result) -> result/1

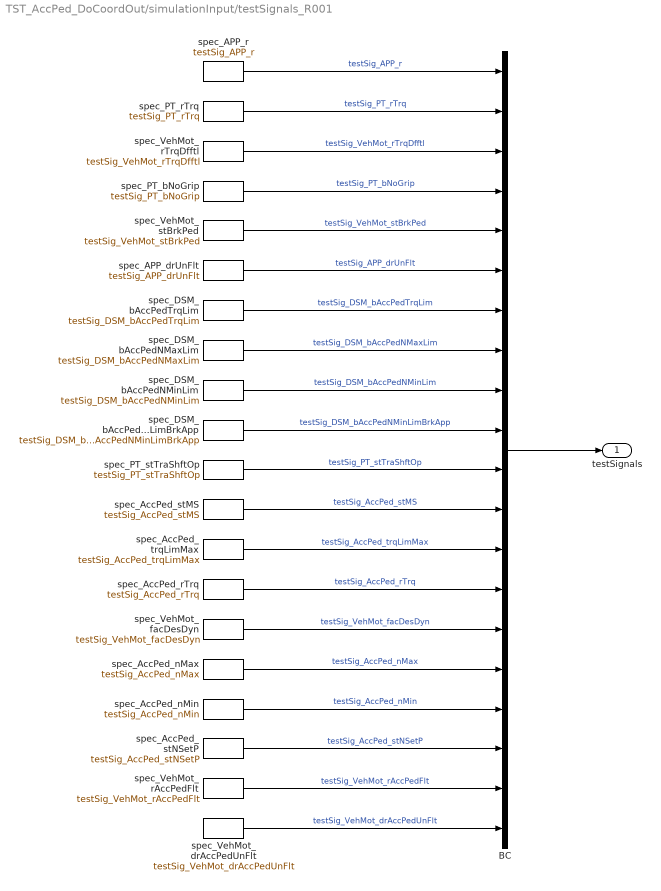
== system TST_AccPed_DoCoordOut/simulationInput/testSignals_R001 ==
  BC : BusCreator  Inputs=20
  spec_APP_drUnFlt : FromWorkspace  VariableName=testSig_APP_drUnFlt  Interpolate=off  OutputAfterFinalValue=Holding final value
  spec_APP_r : FromWorkspace  VariableName=testSig_APP_r  Interpolate=off  OutputAfterFinalValue=Holding final value
  spec_AccPed_nMax : FromWorkspace  VariableName=testSig_AccPed_nMax  Interpolate=off  OutputAfterFinalValue=Holding final value
  spec_AccPed_nMin : FromWorkspace  VariableName=testSig_AccPed_nMin  Interpolate=off  OutputAfterFinalValue=Holding final value
  spec_AccPed_rTrq : FromWorkspace  VariableName=testSig_AccPed_rTrq  Interpolate=off  OutputAfterFinalValue=Holding final value
  spec_AccPed_stMS : FromWorkspace  VariableName=testSig_AccPed_stMS  Interpolate=off  OutputAfterFinalValue=Holding final value
  spec_AccPed_stNSetP : FromWorkspace  VariableName=testSig_AccPed_stNSetP  Interpolate=off  OutputAfterFinalValue=Holding final value
  spec_AccPed_trqLimMax : FromWorkspace  VariableName=testSig_AccPed_trqLimMax  Interpolate=off  OutputAfterFinalValue=Holding final value
  spec_DSM_bAccPedNMaxLim : FromWorkspace  VariableName=testSig_DSM_bAccPedNMaxLim  Interpolate=off  OutputAfterFinalValue=Holding final value
  spec_DSM_bAccPedNMinLim : FromWorkspace  VariableName=testSig_DSM_bAccPedNMinLim  Interpolate=off  OutputAfterFinalValue=Holding final value
  spec_DSM_bAccPedNMinLimBrkApp : FromWorkspace  VariableName=testSig_DSM_bAccPedNMinLimBrkApp  Interpolate=off  OutputAfterFinalValue=Holding final value
  spec_DSM_bAccPedTrqLim : FromWorkspace  VariableName=testSig_DSM_bAccPedTrqLim  Interpolate=off  OutputAfterFinalValue=Holding final value
  spec_PT_bNoGrip : FromWorkspace  VariableName=testSig_PT_bNoGrip  Interpolate=off  OutputAfterFinalValue=Holding final value
  spec_PT_rTrq : FromWorkspace  VariableName=testSig_PT_rTrq  Interpolate=off  OutputAfterFinalValue=Holding final value
  spec_PT_stTraShftOp : FromWorkspace  VariableName=testSig_PT_stTraShftOp  Interpolate=off  OutputAfterFinalValue=Holding final value
  spec_VehMot_drAccPedUnFlt : FromWorkspace  VariableName=testSig_VehMot_drAccPedUnFlt  Interpolate=off  OutputAfterFinalValue=Holding final value
  spec_VehMot_facDesDyn : FromWorkspace  VariableName=testSig_VehMot_facDesDyn  Interpolate=off  OutputAfterFinalValue=Holding final value
  spec_VehMot_rAccPedFlt : FromWorkspace  VariableName=testSig_VehMot_rAccPedFlt  Interpolate=off  OutputAfterFinalValue=Holding final value
  spec_VehMot_rTrqDfftl : FromWorkspace  VariableName=testSig_VehMot_rTrqDfftl  Interpolate=off  OutputAfterFinalValue=Holding final value
  spec_VehMot_stBrkPed : FromWorkspace  VariableName=testSig_VehMot_stBrkPed  Interpolate=off  OutputAfterFinalValue=Holding final value
  testSignals : Outport
  wires:
  BC/1 -> testSignals/1
  spec_APP_r/1 -> BC/1  "testSig_APP_r"
  spec_PT_rTrq/1 -> BC/2  "testSig_PT_rTrq"
  spec_VehMot_rTrqDfftl/1 -> BC/3  "testSig_VehMot_rTrqDfftl"
  spec_PT_bNoGrip/1 -> BC/4  "testSig_PT_bNoGrip"
  spec_VehMot_stBrkPed/1 -> BC/5  "testSig_VehMot_stBrkPed"
  spec_APP_drUnFlt/1 -> BC/6  "testSig_APP_drUnFlt"
  spec_DSM_bAccPedTrqLim/1 -> BC/7  "testSig_DSM_bAccPedTrqLim"
  spec_DSM_bAccPedNMaxLim/1 -> BC/8  "testSig_DSM_bAccPedNMaxLim"
  spec_DSM_bAccPedNMinLim/1 -> BC/9  "testSig_DSM_bAccPedNMinLim"
  spec_DSM_bAccPedNMinLimBrkApp/1 -> BC/10  "testSig_DSM_bAccPedNMinLimBrkApp"
  spec_PT_stTraShftOp/1 -> BC/11  "testSig_PT_stTraShftOp"
  spec_AccPed_stMS/1 -> BC/12  "testSig_AccPed_stMS"
  spec_AccPed_trqLimMax/1 -> BC/13  "testSig_AccPed_trqLimMax"
  spec_AccPed_rTrq/1 -> BC/14  "testSig_AccPed_rTrq"
  spec_VehMot_facDesDyn/1 -> BC/15  "testSig_VehMot_facDesDyn"
  spec_AccPed_nMax/1 -> BC/16  "testSig_AccPed_nMax"
  spec_AccPed_nMin/1 -> BC/17  "testSig_AccPed_nMin"
  spec_AccPed_stNSetP/1 -> BC/18  "testSig_AccPed_stNSetP"
  spec_VehMot_rAccPedFlt/1 -> BC/19  "testSig_VehMot_rAccPedFlt"
  spec_VehMot_drAccPedUnFlt/1 -> BC/20  "testSig_VehMot_drAccPedUnFlt"

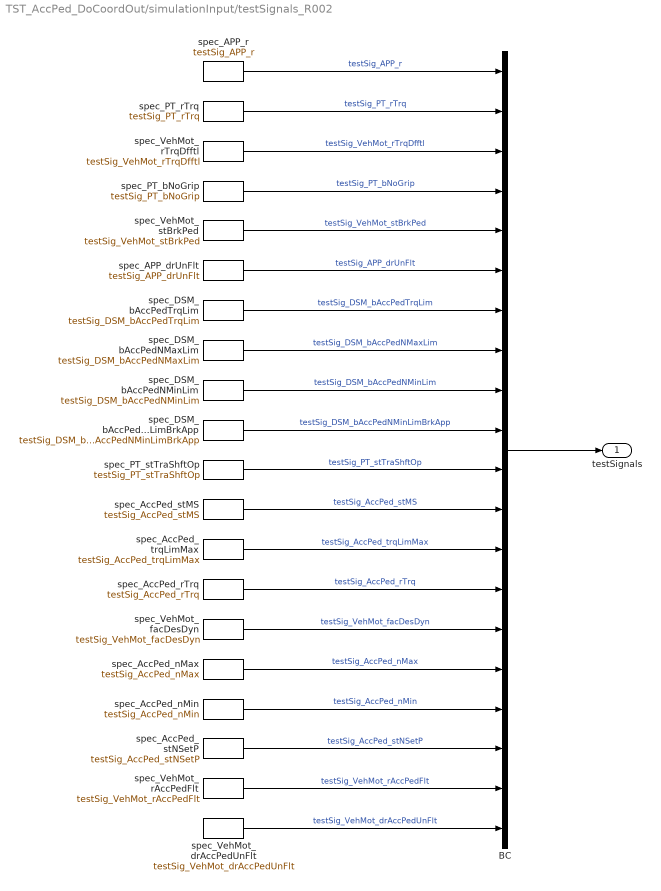
== system TST_AccPed_DoCoordOut/simulationInput/testSignals_R002 ==
  BC : BusCreator  Inputs=20
  spec_APP_drUnFlt : FromWorkspace  VariableName=testSig_APP_drUnFlt  Interpolate=off  OutputAfterFinalValue=Holding final value
  spec_APP_r : FromWorkspace  VariableName=testSig_APP_r  Interpolate=off  OutputAfterFinalValue=Holding final value
  spec_AccPed_nMax : FromWorkspace  VariableName=testSig_AccPed_nMax  Interpolate=off  OutputAfterFinalValue=Holding final value
  spec_AccPed_nMin : FromWorkspace  VariableName=testSig_AccPed_nMin  Interpolate=off  OutputAfterFinalValue=Holding final value
  spec_AccPed_rTrq : FromWorkspace  VariableName=testSig_AccPed_rTrq  Interpolate=off  OutputAfterFinalValue=Holding final value
  spec_AccPed_stMS : FromWorkspace  VariableName=testSig_AccPed_stMS  Interpolate=off  OutputAfterFinalValue=Holding final value
  spec_AccPed_stNSetP : FromWorkspace  VariableName=testSig_AccPed_stNSetP  Interpolate=off  OutputAfterFinalValue=Holding final value
  spec_AccPed_trqLimMax : FromWorkspace  VariableName=testSig_AccPed_trqLimMax  Interpolate=off  OutputAfterFinalValue=Holding final value
  spec_DSM_bAccPedNMaxLim : FromWorkspace  VariableName=testSig_DSM_bAccPedNMaxLim  Interpolate=off  OutputAfterFinalValue=Holding final value
  spec_DSM_bAccPedNMinLim : FromWorkspace  VariableName=testSig_DSM_bAccPedNMinLim  Interpolate=off  OutputAfterFinalValue=Holding final value
  spec_DSM_bAccPedNMinLimBrkApp : FromWorkspace  VariableName=testSig_DSM_bAccPedNMinLimBrkApp  Interpolate=off  OutputAfterFinalValue=Holding final value
  spec_DSM_bAccPedTrqLim : FromWorkspace  VariableName=testSig_DSM_bAccPedTrqLim  Interpolate=off  OutputAfterFinalValue=Holding final value
  spec_PT_bNoGrip : FromWorkspace  VariableName=testSig_PT_bNoGrip  Interpolate=off  OutputAfterFinalValue=Holding final value
  spec_PT_rTrq : FromWorkspace  VariableName=testSig_PT_rTrq  Interpolate=off  OutputAfterFinalValue=Holding final value
  spec_PT_stTraShftOp : FromWorkspace  VariableName=testSig_PT_stTraShftOp  Interpolate=off  OutputAfterFinalValue=Holding final value
  spec_VehMot_drAccPedUnFlt : FromWorkspace  VariableName=testSig_VehMot_drAccPedUnFlt  Interpolate=off  OutputAfterFinalValue=Holding final value
  spec_VehMot_facDesDyn : FromWorkspace  VariableName=testSig_VehMot_facDesDyn  Interpolate=off  OutputAfterFinalValue=Holding final value
  spec_VehMot_rAccPedFlt : FromWorkspace  VariableName=testSig_VehMot_rAccPedFlt  Interpolate=off  OutputAfterFinalValue=Holding final value
  spec_VehMot_rTrqDfftl : FromWorkspace  VariableName=testSig_VehMot_rTrqDfftl  Interpolate=off  OutputAfterFinalValue=Holding final value
  spec_VehMot_stBrkPed : FromWorkspace  VariableName=testSig_VehMot_stBrkPed  Interpolate=off  OutputAfterFinalValue=Holding final value
  testSignals : Outport
  wires:
  BC/1 -> testSignals/1
  spec_APP_r/1 -> BC/1  "testSig_APP_r"
  spec_PT_rTrq/1 -> BC/2  "testSig_PT_rTrq"
  spec_VehMot_rTrqDfftl/1 -> BC/3  "testSig_VehMot_rTrqDfftl"
  spec_PT_bNoGrip/1 -> BC/4  "testSig_PT_bNoGrip"
  spec_VehMot_stBrkPed/1 -> BC/5  "testSig_VehMot_stBrkPed"
  spec_APP_drUnFlt/1 -> BC/6  "testSig_APP_drUnFlt"
  spec_DSM_bAccPedTrqLim/1 -> BC/7  "testSig_DSM_bAccPedTrqLim"
  spec_DSM_bAccPedNMaxLim/1 -> BC/8  "testSig_DSM_bAccPedNMaxLim"
  spec_DSM_bAccPedNMinLim/1 -> BC/9  "testSig_DSM_bAccPedNMinLim"
  spec_DSM_bAccPedNMinLimBrkApp/1 -> BC/10  "testSig_DSM_bAccPedNMinLimBrkApp"
  spec_PT_stTraShftOp/1 -> BC/11  "testSig_PT_stTraShftOp"
  spec_AccPed_stMS/1 -> BC/12  "testSig_AccPed_stMS"
  spec_AccPed_trqLimMax/1 -> BC/13  "testSig_AccPed_trqLimMax"
  spec_AccPed_rTrq/1 -> BC/14  "testSig_AccPed_rTrq"
  spec_VehMot_facDesDyn/1 -> BC/15  "testSig_VehMot_facDesDyn"
  spec_AccPed_nMax/1 -> BC/16  "testSig_AccPed_nMax"
  spec_AccPed_nMin/1 -> BC/17  "testSig_AccPed_nMin"
  spec_AccPed_stNSetP/1 -> BC/18  "testSig_AccPed_stNSetP"
  spec_VehMot_rAccPedFlt/1 -> BC/19  "testSig_VehMot_rAccPedFlt"
  spec_VehMot_drAccPedUnFlt/1 -> BC/20  "testSig_VehMot_drAccPedUnFlt"

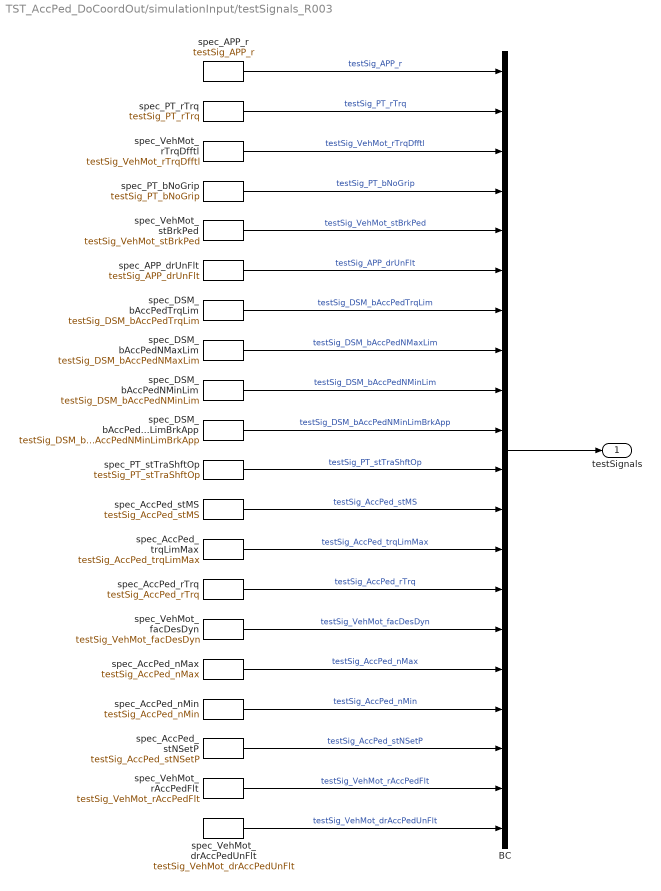
== system TST_AccPed_DoCoordOut/simulationInput/testSignals_R003 ==
  BC : BusCreator  Inputs=20
  spec_APP_drUnFlt : FromWorkspace  VariableName=testSig_APP_drUnFlt  Interpolate=off  OutputAfterFinalValue=Holding final value
  spec_APP_r : FromWorkspace  VariableName=testSig_APP_r  Interpolate=off  OutputAfterFinalValue=Holding final value
  spec_AccPed_nMax : FromWorkspace  VariableName=testSig_AccPed_nMax  Interpolate=off  OutputAfterFinalValue=Holding final value
  spec_AccPed_nMin : FromWorkspace  VariableName=testSig_AccPed_nMin  Interpolate=off  OutputAfterFinalValue=Holding final value
  spec_AccPed_rTrq : FromWorkspace  VariableName=testSig_AccPed_rTrq  Interpolate=off  OutputAfterFinalValue=Holding final value
  spec_AccPed_stMS : FromWorkspace  VariableName=testSig_AccPed_stMS  Interpolate=off  OutputAfterFinalValue=Holding final value
  spec_AccPed_stNSetP : FromWorkspace  VariableName=testSig_AccPed_stNSetP  Interpolate=off  OutputAfterFinalValue=Holding final value
  spec_AccPed_trqLimMax : FromWorkspace  VariableName=testSig_AccPed_trqLimMax  Interpolate=off  OutputAfterFinalValue=Holding final value
  spec_DSM_bAccPedNMaxLim : FromWorkspace  VariableName=testSig_DSM_bAccPedNMaxLim  Interpolate=off  OutputAfterFinalValue=Holding final value
  spec_DSM_bAccPedNMinLim : FromWorkspace  VariableName=testSig_DSM_bAccPedNMinLim  Interpolate=off  OutputAfterFinalValue=Holding final value
  spec_DSM_bAccPedNMinLimBrkApp : FromWorkspace  VariableName=testSig_DSM_bAccPedNMinLimBrkApp  Interpolate=off  OutputAfterFinalValue=Holding final value
  spec_DSM_bAccPedTrqLim : FromWorkspace  VariableName=testSig_DSM_bAccPedTrqLim  Interpolate=off  OutputAfterFinalValue=Holding final value
  spec_PT_bNoGrip : FromWorkspace  VariableName=testSig_PT_bNoGrip  Interpolate=off  OutputAfterFinalValue=Holding final value
  spec_PT_rTrq : FromWorkspace  VariableName=testSig_PT_rTrq  Interpolate=off  OutputAfterFinalValue=Holding final value
  spec_PT_stTraShftOp : FromWorkspace  VariableName=testSig_PT_stTraShftOp  Interpolate=off  OutputAfterFinalValue=Holding final value
  spec_VehMot_drAccPedUnFlt : FromWorkspace  VariableName=testSig_VehMot_drAccPedUnFlt  Interpolate=off  OutputAfterFinalValue=Holding final value
  spec_VehMot_facDesDyn : FromWorkspace  VariableName=testSig_VehMot_facDesDyn  Interpolate=off  OutputAfterFinalValue=Holding final value
  spec_VehMot_rAccPedFlt : FromWorkspace  VariableName=testSig_VehMot_rAccPedFlt  Interpolate=off  OutputAfterFinalValue=Holding final value
  spec_VehMot_rTrqDfftl : FromWorkspace  VariableName=testSig_VehMot_rTrqDfftl  Interpolate=off  OutputAfterFinalValue=Holding final value
  spec_VehMot_stBrkPed : FromWorkspace  VariableName=testSig_VehMot_stBrkPed  Interpolate=off  OutputAfterFinalValue=Holding final value
  testSignals : Outport
  wires:
  BC/1 -> testSignals/1
  spec_APP_r/1 -> BC/1  "testSig_APP_r"
  spec_PT_rTrq/1 -> BC/2  "testSig_PT_rTrq"
  spec_VehMot_rTrqDfftl/1 -> BC/3  "testSig_VehMot_rTrqDfftl"
  spec_PT_bNoGrip/1 -> BC/4  "testSig_PT_bNoGrip"
  spec_VehMot_stBrkPed/1 -> BC/5  "testSig_VehMot_stBrkPed"
  spec_APP_drUnFlt/1 -> BC/6  "testSig_APP_drUnFlt"
  spec_DSM_bAccPedTrqLim/1 -> BC/7  "testSig_DSM_bAccPedTrqLim"
  spec_DSM_bAccPedNMaxLim/1 -> BC/8  "testSig_DSM_bAccPedNMaxLim"
  spec_DSM_bAccPedNMinLim/1 -> BC/9  "testSig_DSM_bAccPedNMinLim"
  spec_DSM_bAccPedNMinLimBrkApp/1 -> BC/10  "testSig_DSM_bAccPedNMinLimBrkApp"
  spec_PT_stTraShftOp/1 -> BC/11  "testSig_PT_stTraShftOp"
  spec_AccPed_stMS/1 -> BC/12  "testSig_AccPed_stMS"
  spec_AccPed_trqLimMax/1 -> BC/13  "testSig_AccPed_trqLimMax"
  spec_AccPed_rTrq/1 -> BC/14  "testSig_AccPed_rTrq"
  spec_VehMot_facDesDyn/1 -> BC/15  "testSig_VehMot_facDesDyn"
  spec_AccPed_nMax/1 -> BC/16  "testSig_AccPed_nMax"
  spec_AccPed_nMin/1 -> BC/17  "testSig_AccPed_nMin"
  spec_AccPed_stNSetP/1 -> BC/18  "testSig_AccPed_stNSetP"
  spec_VehMot_rAccPedFlt/1 -> BC/19  "testSig_VehMot_rAccPedFlt"
  spec_VehMot_drAccPedUnFlt/1 -> BC/20  "testSig_VehMot_drAccPedUnFlt"

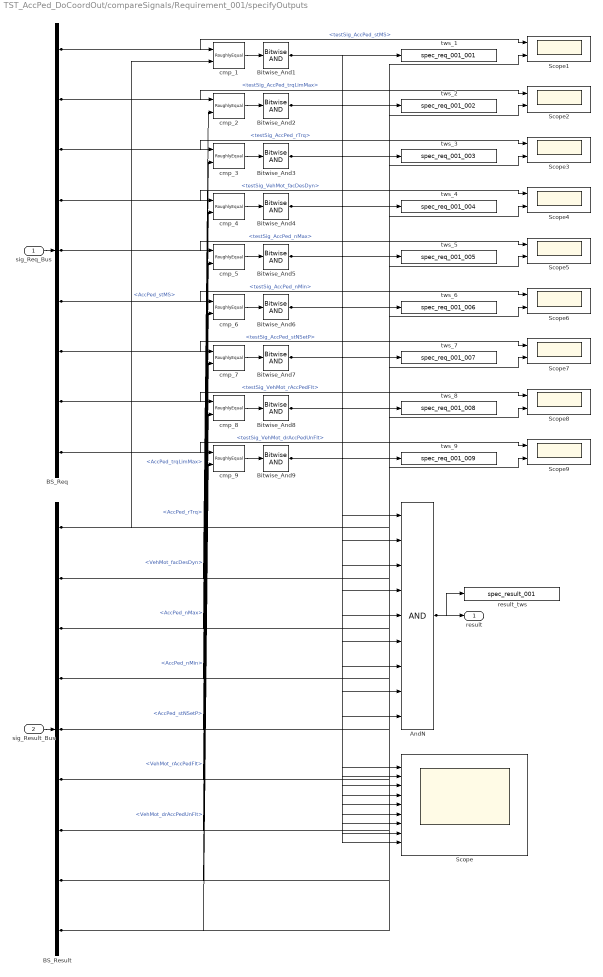
== system TST_AccPed_DoCoordOut/compareSignals/Requirement_001/specifyOutputs ==
  sig_Req_Bus : Inport
  sig_Result_Bus : Inport  Port=2
  AndN : Logic  Inputs=9
  BS_Req : BusSelector  OutputSignals=testSig_AccPed_stMS,testSig_AccPed_trqLimMax,testSig_AccPed_rTrq,testSig_VehMot_facDesDyn,testSig_AccPed_nMax,testSig_AccPed_nMin,testSig_AccPed_stNSetP,testSig_VehMot_rAccPedFlt,testSig_VehMot_drAccPedUnFlt
  BS_Result : BusSelector  OutputSignals=AccPed_stMS,AccPed_trqLimMax,AccPed_rTrq,VehMot_facDesDyn,AccPed_nMax,AccPed_nMin,AccPed_stNSetP,VehMot_rAccPedFlt,VehMot_drAccPedUnFlt
  Bitwise_And{1..9} (9 alike) : simulink/Logic and Bit Operations/Bitwise Operator  logicop=AND  UseBitMask=off  BitMask=bin2dec('11011001')  BitMaskRealWorld=Stored Integer
  Scope : Scope  NumInputPorts=9
  Scope{1..9} (9 alike) : Scope  NumInputPorts=2
  cmp_{1..9} (9 alike) : UnitTest_Lib/RoughlyEqual  slope=0.1
  result_tws : ToWorkspace  VariableName=spec_result_001
  tws_1 : ToWorkspace  VariableName=spec_req_001_001
  tws_2 : ToWorkspace  VariableName=spec_req_001_002
  tws_3 : ToWorkspace  VariableName=spec_req_001_003
  tws_4 : ToWorkspace  VariableName=spec_req_001_004
  tws_5 : ToWorkspace  VariableName=spec_req_001_005
  tws_6 : ToWorkspace  VariableName=spec_req_001_006
  tws_7 : ToWorkspace  VariableName=spec_req_001_007
  tws_8 : ToWorkspace  VariableName=spec_req_001_008
  tws_9 : ToWorkspace  VariableName=spec_req_001_009
  result : Outport
  wires:
  sig_Req_Bus/1 -> BS_Req/1
  sig_Result_Bus/1 -> BS_Result/1
  AndN/1 -> result/1, result_tws/1
  BS_Req/1 -> cmp_1/1, Scope1/1  "<testSig_AccPed_stMS>"
  BS_Result/1 -> cmp_1/2, Scope1/2  "<AccPed_stMS>"
  cmp_1/1 -> Bitwise_And1/1
  Bitwise_And1/1 -> tws_1/1, AndN/1, Scope/1
  BS_Req/2 -> cmp_2/1, Scope2/1  "<testSig_AccPed_trqLimMax>"
  BS_Result/2 -> cmp_2/2, Scope2/2  "<AccPed_trqLimMax>"
  cmp_2/1 -> Bitwise_And2/1
  Bitwise_And2/1 -> tws_2/1, AndN/2, Scope/2
  BS_Req/3 -> cmp_3/1, Scope3/1  "<testSig_AccPed_rTrq>"
  BS_Result/3 -> cmp_3/2, Scope3/2  "<AccPed_rTrq>"
  cmp_3/1 -> Bitwise_And3/1
  Bitwise_And3/1 -> tws_3/1, AndN/3, Scope/3
  BS_Req/4 -> cmp_4/1, Scope4/1  "<testSig_VehMot_facDesDyn>"
  BS_Result/4 -> cmp_4/2, Scope4/2  "<VehMot_facDesDyn>"
  cmp_4/1 -> Bitwise_And4/1
  Bitwise_And4/1 -> tws_4/1, AndN/4, Scope/4
  BS_Req/5 -> cmp_5/1, Scope5/1  "<testSig_AccPed_nMax>"
  BS_Result/5 -> cmp_5/2, Scope5/2  "<AccPed_nMax>"
  cmp_5/1 -> Bitwise_And5/1
  Bitwise_And5/1 -> tws_5/1, AndN/5, Scope/5
  BS_Req/6 -> cmp_6/1, Scope6/1  "<testSig_AccPed_nMin>"
  BS_Result/6 -> cmp_6/2, Scope6/2  "<AccPed_nMin>"
  cmp_6/1 -> Bitwise_And6/1
  Bitwise_And6/1 -> tws_6/1, AndN/6, Scope/6
  BS_Req/7 -> cmp_7/1, Scope7/1  "<testSig_AccPed_stNSetP>"
  BS_Result/7 -> cmp_7/2, Scope7/2  "<AccPed_stNSetP>"
  cmp_7/1 -> Bitwise_And7/1
  Bitwise_And7/1 -> tws_7/1, AndN/7, Scope/7
  BS_Req/8 -> cmp_8/1, Scope8/1  "<testSig_VehMot_rAccPedFlt>"
  BS_Result/8 -> cmp_8/2, Scope8/2  "<VehMot_rAccPedFlt>"
  cmp_8/1 -> Bitwise_And8/1
  Bitwise_And8/1 -> tws_8/1, AndN/8, Scope/8
  BS_Req/9 -> cmp_9/1, Scope9/1  "<testSig_VehMot_drAccPedUnFlt>"
  BS_Result/9 -> cmp_9/2, Scope9/2  "<VehMot_drAccPedUnFlt>"
  cmp_9/1 -> Bitwise_And9/1
  Bitwise_And9/1 -> tws_9/1, AndN/9, Scope/9

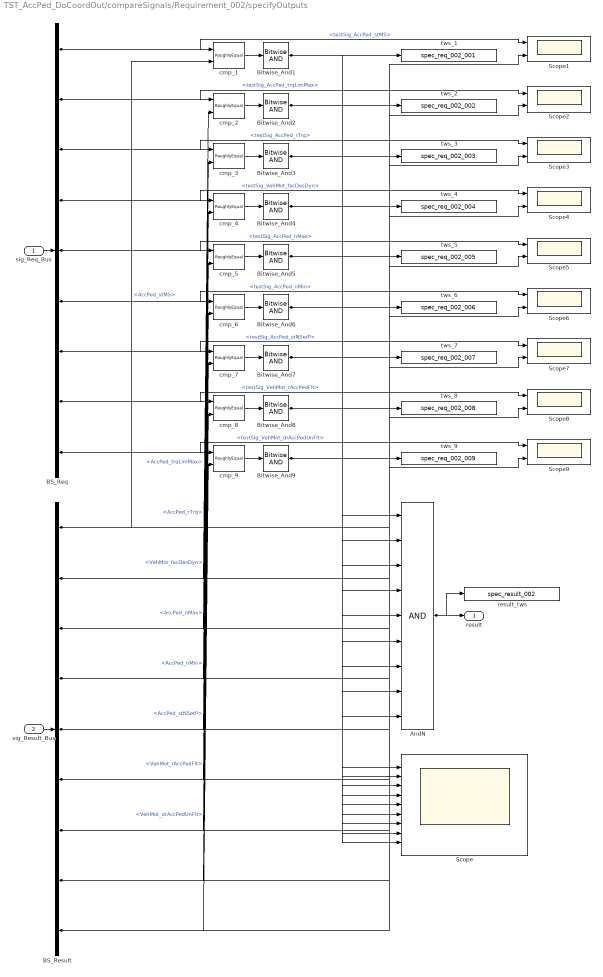
== system TST_AccPed_DoCoordOut/compareSignals/Requirement_002/specifyOutputs ==
  sig_Req_Bus : Inport
  sig_Result_Bus : Inport  Port=2
  AndN : Logic  Inputs=9
  BS_Req : BusSelector  OutputSignals=testSig_AccPed_stMS,testSig_AccPed_trqLimMax,testSig_AccPed_rTrq,testSig_VehMot_facDesDyn,testSig_AccPed_nMax,testSig_AccPed_nMin,testSig_AccPed_stNSetP,testSig_VehMot_rAccPedFlt,testSig_VehMot_drAccPedUnFlt
  BS_Result : BusSelector  OutputSignals=AccPed_stMS,AccPed_trqLimMax,AccPed_rTrq,VehMot_facDesDyn,AccPed_nMax,AccPed_nMin,AccPed_stNSetP,VehMot_rAccPedFlt,VehMot_drAccPedUnFlt
  Bitwise_And{1..9} (9 alike) : simulink/Logic and Bit Operations/Bitwise Operator  logicop=AND  UseBitMask=off  BitMask=bin2dec('11011001')  BitMaskRealWorld=Stored Integer
  Scope : Scope  NumInputPorts=9
  Scope{1..9} (9 alike) : Scope  NumInputPorts=2
  cmp_{1..9} (9 alike) : UnitTest_Lib/RoughlyEqual  slope=0.1
  result_tws : ToWorkspace  VariableName=spec_result_002
  tws_1 : ToWorkspace  VariableName=spec_req_002_001
  tws_2 : ToWorkspace  VariableName=spec_req_002_002
  tws_3 : ToWorkspace  VariableName=spec_req_002_003
  tws_4 : ToWorkspace  VariableName=spec_req_002_004
  tws_5 : ToWorkspace  VariableName=spec_req_002_005
  tws_6 : ToWorkspace  VariableName=spec_req_002_006
  tws_7 : ToWorkspace  VariableName=spec_req_002_007
  tws_8 : ToWorkspace  VariableName=spec_req_002_008
  tws_9 : ToWorkspace  VariableName=spec_req_002_009
  result : Outport
  wires:
  sig_Req_Bus/1 -> BS_Req/1
  sig_Result_Bus/1 -> BS_Result/1
  AndN/1 -> result/1, result_tws/1
  BS_Req/1 -> cmp_1/1, Scope1/1  "<testSig_AccPed_stMS>"
  BS_Result/1 -> cmp_1/2, Scope1/2  "<AccPed_stMS>"
  cmp_1/1 -> Bitwise_And1/1
  Bitwise_And1/1 -> tws_1/1, AndN/1, Scope/1
  BS_Req/2 -> cmp_2/1, Scope2/1  "<testSig_AccPed_trqLimMax>"
  BS_Result/2 -> cmp_2/2, Scope2/2  "<AccPed_trqLimMax>"
  cmp_2/1 -> Bitwise_And2/1
  Bitwise_And2/1 -> tws_2/1, AndN/2, Scope/2
  BS_Req/3 -> cmp_3/1, Scope3/1  "<testSig_AccPed_rTrq>"
  BS_Result/3 -> cmp_3/2, Scope3/2  "<AccPed_rTrq>"
  cmp_3/1 -> Bitwise_And3/1
  Bitwise_And3/1 -> tws_3/1, AndN/3, Scope/3
  BS_Req/4 -> cmp_4/1, Scope4/1  "<testSig_VehMot_facDesDyn>"
  BS_Result/4 -> cmp_4/2, Scope4/2  "<VehMot_facDesDyn>"
  cmp_4/1 -> Bitwise_And4/1
  Bitwise_And4/1 -> tws_4/1, AndN/4, Scope/4
  BS_Req/5 -> cmp_5/1, Scope5/1  "<testSig_AccPed_nMax>"
  BS_Result/5 -> cmp_5/2, Scope5/2  "<AccPed_nMax>"
  cmp_5/1 -> Bitwise_And5/1
  Bitwise_And5/1 -> tws_5/1, AndN/5, Scope/5
  BS_Req/6 -> cmp_6/1, Scope6/1  "<testSig_AccPed_nMin>"
  BS_Result/6 -> cmp_6/2, Scope6/2  "<AccPed_nMin>"
  cmp_6/1 -> Bitwise_And6/1
  Bitwise_And6/1 -> tws_6/1, AndN/6, Scope/6
  BS_Req/7 -> cmp_7/1, Scope7/1  "<testSig_AccPed_stNSetP>"
  BS_Result/7 -> cmp_7/2, Scope7/2  "<AccPed_stNSetP>"
  cmp_7/1 -> Bitwise_And7/1
  Bitwise_And7/1 -> tws_7/1, AndN/7, Scope/7
  BS_Req/8 -> cmp_8/1, Scope8/1  "<testSig_VehMot_rAccPedFlt>"
  BS_Result/8 -> cmp_8/2, Scope8/2  "<VehMot_rAccPedFlt>"
  cmp_8/1 -> Bitwise_And8/1
  Bitwise_And8/1 -> tws_8/1, AndN/8, Scope/8
  BS_Req/9 -> cmp_9/1, Scope9/1  "<testSig_VehMot_drAccPedUnFlt>"
  BS_Result/9 -> cmp_9/2, Scope9/2  "<VehMot_drAccPedUnFlt>"
  cmp_9/1 -> Bitwise_And9/1
  Bitwise_And9/1 -> tws_9/1, AndN/9, Scope/9

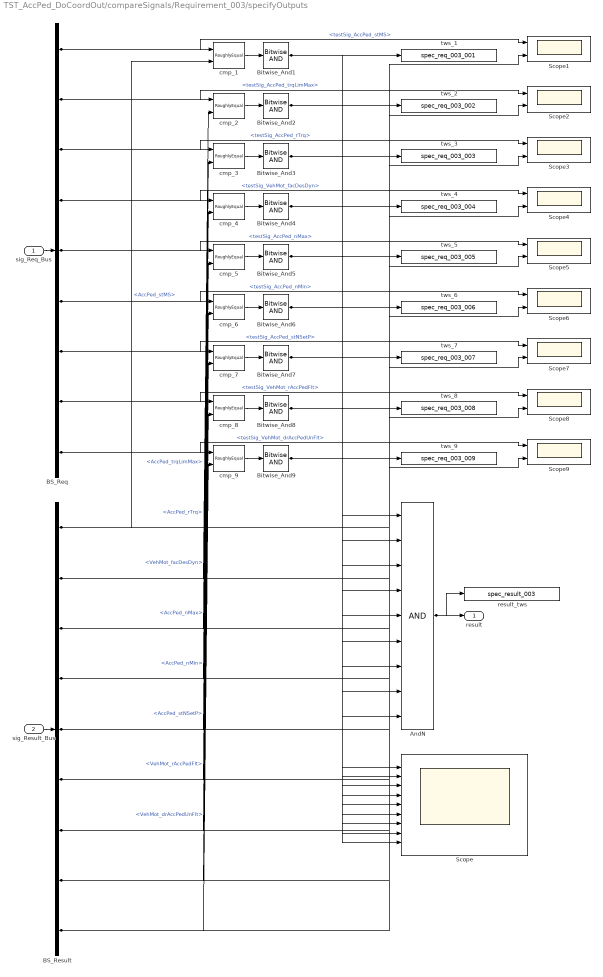
== system TST_AccPed_DoCoordOut/compareSignals/Requirement_003/specifyOutputs ==
  sig_Req_Bus : Inport
  sig_Result_Bus : Inport  Port=2
  AndN : Logic  Inputs=9
  BS_Req : BusSelector  OutputSignals=testSig_AccPed_stMS,testSig_AccPed_trqLimMax,testSig_AccPed_rTrq,testSig_VehMot_facDesDyn,testSig_AccPed_nMax,testSig_AccPed_nMin,testSig_AccPed_stNSetP,testSig_VehMot_rAccPedFlt,testSig_VehMot_drAccPedUnFlt
  BS_Result : BusSelector  OutputSignals=AccPed_stMS,AccPed_trqLimMax,AccPed_rTrq,VehMot_facDesDyn,AccPed_nMax,AccPed_nMin,AccPed_stNSetP,VehMot_rAccPedFlt,VehMot_drAccPedUnFlt
  Bitwise_And{1..9} (9 alike) : simulink/Logic and Bit Operations/Bitwise Operator  logicop=AND  UseBitMask=off  BitMask=bin2dec('11011001')  BitMaskRealWorld=Stored Integer
  Scope : Scope  NumInputPorts=9
  Scope{1..9} (9 alike) : Scope  NumInputPorts=2
  cmp_{1..9} (9 alike) : UnitTest_Lib/RoughlyEqual  slope=0.1
  result_tws : ToWorkspace  VariableName=spec_result_003
  tws_1 : ToWorkspace  VariableName=spec_req_003_001
  tws_2 : ToWorkspace  VariableName=spec_req_003_002
  tws_3 : ToWorkspace  VariableName=spec_req_003_003
  tws_4 : ToWorkspace  VariableName=spec_req_003_004
  tws_5 : ToWorkspace  VariableName=spec_req_003_005
  tws_6 : ToWorkspace  VariableName=spec_req_003_006
  tws_7 : ToWorkspace  VariableName=spec_req_003_007
  tws_8 : ToWorkspace  VariableName=spec_req_003_008
  tws_9 : ToWorkspace  VariableName=spec_req_003_009
  result : Outport
  wires:
  sig_Req_Bus/1 -> BS_Req/1
  sig_Result_Bus/1 -> BS_Result/1
  AndN/1 -> result/1, result_tws/1
  BS_Req/1 -> cmp_1/1, Scope1/1  "<testSig_AccPed_stMS>"
  BS_Result/1 -> cmp_1/2, Scope1/2  "<AccPed_stMS>"
  cmp_1/1 -> Bitwise_And1/1
  Bitwise_And1/1 -> tws_1/1, AndN/1, Scope/1
  BS_Req/2 -> cmp_2/1, Scope2/1  "<testSig_AccPed_trqLimMax>"
  BS_Result/2 -> cmp_2/2, Scope2/2  "<AccPed_trqLimMax>"
  cmp_2/1 -> Bitwise_And2/1
  Bitwise_And2/1 -> tws_2/1, AndN/2, Scope/2
  BS_Req/3 -> cmp_3/1, Scope3/1  "<testSig_AccPed_rTrq>"
  BS_Result/3 -> cmp_3/2, Scope3/2  "<AccPed_rTrq>"
  cmp_3/1 -> Bitwise_And3/1
  Bitwise_And3/1 -> tws_3/1, AndN/3, Scope/3
  BS_Req/4 -> cmp_4/1, Scope4/1  "<testSig_VehMot_facDesDyn>"
  BS_Result/4 -> cmp_4/2, Scope4/2  "<VehMot_facDesDyn>"
  cmp_4/1 -> Bitwise_And4/1
  Bitwise_And4/1 -> tws_4/1, AndN/4, Scope/4
  BS_Req/5 -> cmp_5/1, Scope5/1  "<testSig_AccPed_nMax>"
  BS_Result/5 -> cmp_5/2, Scope5/2  "<AccPed_nMax>"
  cmp_5/1 -> Bitwise_And5/1
  Bitwise_And5/1 -> tws_5/1, AndN/5, Scope/5
  BS_Req/6 -> cmp_6/1, Scope6/1  "<testSig_AccPed_nMin>"
  BS_Result/6 -> cmp_6/2, Scope6/2  "<AccPed_nMin>"
  cmp_6/1 -> Bitwise_And6/1
  Bitwise_And6/1 -> tws_6/1, AndN/6, Scope/6
  BS_Req/7 -> cmp_7/1, Scope7/1  "<testSig_AccPed_stNSetP>"
  BS_Result/7 -> cmp_7/2, Scope7/2  "<AccPed_stNSetP>"
  cmp_7/1 -> Bitwise_And7/1
  Bitwise_And7/1 -> tws_7/1, AndN/7, Scope/7
  BS_Req/8 -> cmp_8/1, Scope8/1  "<testSig_VehMot_rAccPedFlt>"
  BS_Result/8 -> cmp_8/2, Scope8/2  "<VehMot_rAccPedFlt>"
  cmp_8/1 -> Bitwise_And8/1
  Bitwise_And8/1 -> tws_8/1, AndN/8, Scope/8
  BS_Req/9 -> cmp_9/1, Scope9/1  "<testSig_VehMot_drAccPedUnFlt>"
  BS_Result/9 -> cmp_9/2, Scope9/2  "<VehMot_drAccPedUnFlt>"
  cmp_9/1 -> Bitwise_And9/1
  Bitwise_And9/1 -> tws_9/1, AndN/9, Scope/9
